simulink library "vxlib"  (Simulink 6.0)
PreLoadFcn:
  | warning('''vxlib'' is obsolete, use ''vxlib1'' instead.');
settings Model: Creator=jwu  LastModifiedBy=jcarrick  ExtModeAutoUpdateStatusClock=off

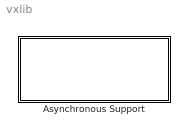
== system vxlib ==
  Asynchronous Support : Subsystem
      mask Display: disp('Asynchronous\nInterrupt\nSupport')

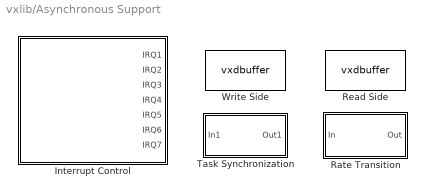
== system vxlib/Asynchronous Support ==
  Interrupt Control : Subsystem  Tag=AsyncRateTransition  mask(VxWorks Interrupt Block){mode=RTW, irqNumbers=[1 2 3 4 5 6 7], irqOffsets=[192 193 194 195 196 197 198], irqPreemptionFlags=[1], irqDirection=Rising}
      mask prompts: irqNumbers "VME interrupt number(s)"; irqOffsets "VME interrupt vector offset number(s)"; irqPreemptionFlags "Preemption flag(s): ISR preemptable-1, non-preemptable-0"; irqDirection "IRQ direction (simulation only)"
      mask help: Install the downstream function-call subsystem as a VME Interrupt Service Routine.
      mask init:
      | if isunix,
      |   devicedir = '/rtw/c/tornado/devices';
      | else,
      |   devicedir = '\rtw\c\tornado\devices';
      | end;
      | 
      | if isempty(findstr(devicedir, path)),
      |   if isempty(getenv('TMW_V5_SANDBOX')),
      |     addpath([matlabroot devicedir]);
      |   else,
      |     addpath([getenv('TMW_V5_SANDBOX') devicedir]);
      |   end;
      | end
      | 
      | if mode == 1
      |   str0 = '';
      |   str1 = 'Interrupt';
      |   str2 = 'Emulation';
      |   str3 = '(Simulation)';
      | elseif mode == 2
      |   str0 = 'VxWorks';
      |   str1 = 'VME Interrupt';
      |   str2 = 'Registration';
      |   str3 = '(RTW)';
      | end;
      | numbers = str2num(irqNumbers);
      | offsets = str2num(irqOffsets);
      | flags = str2num(irqPreemptionFlags);
      | wizardErrTxt = feval('vxintbuild', numbers, offsets, irqDirection, mode, flags);
      | if length(wizardErrTxt)
      |   errordlg(wizardErrTxt, 'Interrupt Block Error', 'modal');
      | end
      mask Help: web(['file://',docroot,'/toolbox/rtw/vxinterrupt.html']);
      mask StyleString: popup(Simulation|RTW),edit,edit,edit,popup(Rising|Falling|Either)
      mask Display:
      | text(.1, .75, str0)
      | text(.1, .60, str1)
      | text(.1, .45, str2)
      | text(.1, .30, str3)
  Rate Transition : Subsystem  mask(Rate Transition){sample_time=-1}
      mask prompts: sample_time "Sample time"
      mask help: Converts rate of input signal to specified sample time.
      mask Help: web(['file://',docroot,'/toolbox/rtw/vxrate.html']);
      mask Display: disp(['Unprotected\nAsynchronous\nRate Transition'])
  Read Side : S-Function  FunctionName=vxdbuffer  Parameters=DB_Type, sample_time  mask(Asynchronous Rate Transition: Reader){sample_time=-1}
      mask prompts: sample_time "Sample time"
      mask help: Double Buffer data between asynchronous subsystems/blocks in a model.
      mask init:
      | if isunix,
      |   devicedir = '/rtw/c/tornado/devices';
      | else,
      |   devicedir = '\rtw\c\tornado\devices';
      | end;
      | 
      | if isempty(findstr(devicedir, path)),
      |   if isempty(getenv('TMW_V5_SANDBOX')),
      |     addpath([matlabroot devicedir]);
      |   else,
      |     addpath([getenv('TMW_V5_SANDBOX') devicedir]);
      |   end;
      | end
      | DB_Type = 'READ';
      mask Help: web(['file://',docroot,'/toolbox/rtw/vxdbuffer.html']);
      mask Display: disp(['Asynchronous\nRate Transition\n(Reader)'])
  Task Synchronization : Subsystem  mask(VxWorks Task Block){taskName=, taskPriority=20, taskStackSize=1024}
      mask prompts: taskName "Task name (optional) (10 characters or less)"; taskPriority "Task priority (0-255)"; taskStackSize "Stack size (bytes)"
      mask help: Spawns the downstream function-call subsystem as a VxWorks task.
      mask init:
      | if isunix,
      |   devicedir = '/rtw/c/tornado/devices';
      | else,
      |   devicedir = '\rtw\c\tornado\devices';
      | end;
      | 
      | if isempty(findstr(devicedir, path)),
      |   if isempty(getenv('TMW_V5_SANDBOX')),
      |     addpath([matlabroot devicedir]);
      |   else,
      |     addpath([getenv('TMW_V5_SANDBOX') devicedir]);
      |   end;
      | end
      | 
      | if ~iscvar(taskName) & (length(taskName) > 0)
      |    errordlg('invalid Task Name, first character must be a letter or underscore and remaining characters must be letters,underscores or numbers.','Task Block Error','replace');
      |    taskName = '';
      | end
      mask Help: web(['file://',docroot,'/toolbox/rtw/vxtask.html']);
      mask Display: disp(['RTW Task\n',taskName])
  Write Side : S-Function  FunctionName=vxdbuffer  Parameters=DB_Type, sample_time  mask(Asynchronous Rate Transition: Writer){sample_time=-1}
      mask prompts: sample_time "Sample time"
      mask help: Double Buffer data between asynchronous subsystems/blocks in a model.
      mask init:
      | if isunix,
      |   devicedir = '/rtw/c/tornado/devices';
      | else,
      |   devicedir = '\rtw\c\tornado\devices';
      | end;
      | 
      | if isempty(findstr(devicedir, path)),
      |   if isempty(getenv('TMW_V5_SANDBOX')),
      |     addpath([matlabroot devicedir]);
      |   else,
      |     addpath([getenv('TMW_V5_SANDBOX') devicedir]);
      |   end;
      | end
      | DB_Type = 'WRITE';
      mask Help: web(['file://',docroot,'/toolbox/rtw/vxdbuffer.html']);
      mask Display: disp(['Asynchronous\nRate Transition\n(Writer)'])

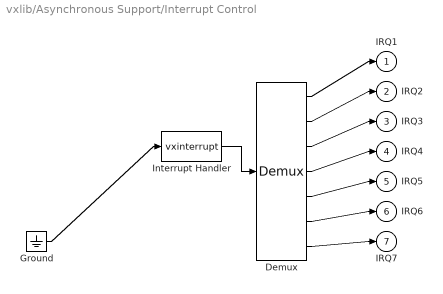
== system vxlib/Asynchronous Support/Interrupt Control ==
  Demux : Demux  Outputs=7
  Ground : Ground
  Interrupt Handler : S-Function  FunctionName=vxinterrupt  Parameters=mode, numbers, offsets, irqDirection, flags
  IRQ1 : Outport
  IRQ2 : Outport  Port=2
  IRQ3 : Outport  Port=3
  IRQ4 : Outport  Port=4
  IRQ5 : Outport  Port=5
  IRQ6 : Outport  Port=6
  IRQ7 : Outport  Port=7
  wires:
  Demux/7 -> IRQ7/1
  Demux/6 -> IRQ6/1
  Demux/5 -> IRQ5/1
  Demux/4 -> IRQ4/1
  Demux/3 -> IRQ3/1
  Demux/2 -> IRQ2/1
  Interrupt Handler/1 -> Demux/1
  Demux/1 -> IRQ1/1
  Ground/1 -> Interrupt Handler/1

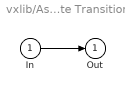
== system vxlib/Asynchronous Support/Rate Transition ==
  In : Inport  Tag=AsyncRateTransition  SampleTime=sample_time
  Out : Outport  Tag=AsyncRateTransition  InitialOutput=0
  wires:
  In/1 -> Out/1

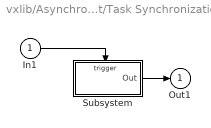
== system vxlib/Asynchronous Support/Task Synchronization ==
  In1 : Inport
  Subsystem : Subsystem  TreatAsAtomicUnit=on
      mask Type: VxWorks Task Block
  Out1 : Outport
  wires:
  In1/1 -> Subsystem/Trigger
  Subsystem/1(Out) -> Out1/1

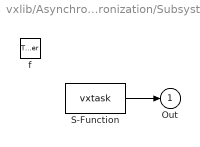
== system vxlib/Asynchronous Support/Task Synchronization/Subsystem ==
  f : TriggerPort  TriggerType=function-call
  S-Function : S-Function  FunctionName=vxtask  Parameters=taskName, taskPriority, taskStackSize
  Out : Outport
  wires:
  S-Function/1 -> Out/1
